simulink model "SF049A_LoaMgr"  (R2013b)
settings: Solver=FixedStepDiscrete  SolverMode=SingleTasking  StartTime=0.0  StopTime=1  FixedStep=0.002  RelTol=1e-3
values from neighbouring files (symbols this model uses):
  CURRMEASLOAMTGTNMASK_CNT_U08 = DataDict.Constant    [SF049A_LoaMgr_DataDict.m]
  IVTRLOAMTGTNMASK_CNT_U08 = DataDict.Constant    [SF049A_LoaMgr_DataDict.m]
  LOAMAXSLEW_ULSPERSEC_F32 = DataDict.Constant    [SF049A_LoaMgr_DataDict.m]
  LoaMgrCurrIvtrMtgtnRate = DataDict.Calibration    [SF049A_LoaMgr_DataDict.m]
  LoaMgrCurrIvtrMtgtnSca = DataDict.Calibration    [SF049A_LoaMgr_DataDict.m]
  LoaMgrCurrIvtrMtgtnScaZeroEna = DataDict.Calibration    [SF049A_LoaMgr_DataDict.m]
  LoaMgrCurrMeasIdptSig0Resp = DataDict.Calibration    [SF049A_LoaMgr_DataDict.m]
  LoaMgrCurrMeasIdptSig1Resp = DataDict.Calibration    [SF049A_LoaMgr_DataDict.m]
  LoaMgrCurrMeasIdptSig2Resp = DataDict.Calibration    [SF049A_LoaMgr_DataDict.m]
  LoaMgrCurrMeasIdptSigFltThd = DataDict.Calibration    [SF049A_LoaMgr_DataDict.m]
  LoaMgrCurrMeasMtgtnRate = DataDict.Calibration    [SF049A_LoaMgr_DataDict.m]
  LoaMgrCurrMeasMtgtnSca = DataDict.Calibration    [SF049A_LoaMgr_DataDict.m]
  LoaMgrCurrMeasMtgtnScaZeroEna = DataDict.Calibration    [SF049A_LoaMgr_DataDict.m]
  LoaMgrFadeOutStRate = DataDict.Calibration    [SF049A_LoaMgr_DataDict.m]
  LoaMgrHwTqIdptSig0NoTqLoaResp = DataDict.Calibration    [SF049A_LoaMgr_DataDict.m]
  LoaMgrHwTqIdptSig1NoTqLoaResp = DataDict.Calibration    [SF049A_LoaMgr_DataDict.m]
  LoaMgrHwTqIdptSig2Resp = DataDict.Calibration    [SF049A_LoaMgr_DataDict.m]
  LoaMgrHwTqIdptSig4Resp = DataDict.Calibration    [SF049A_LoaMgr_DataDict.m]
  LoaMgrHwTqIdptSigFltThd = DataDict.Calibration    [SF049A_LoaMgr_DataDict.m]
  LoaMgrHwTqLoaAvlResp = DataDict.Calibration    [SF049A_LoaMgr_DataDict.m]
  LoaMgrIvtrIdptSig0Resp = DataDict.Calibration    [SF049A_LoaMgr_DataDict.m]
  LoaMgrIvtrIdptSig1Resp = DataDict.Calibration    [SF049A_LoaMgr_DataDict.m]
  LoaMgrIvtrIdptSig2Resp = DataDict.Calibration    [SF049A_LoaMgr_DataDict.m]
  LoaMgrIvtrIdptSigFltThd = DataDict.Calibration    [SF049A_LoaMgr_DataDict.m]
  LoaMgrIvtrMtgtnRate = DataDict.Calibration    [SF049A_LoaMgr_DataDict.m]
  LoaMgrIvtrMtgtnSca = DataDict.Calibration    [SF049A_LoaMgr_DataDict.m]
  LoaMgrIvtrMtgtnScaZeroEna = DataDict.Calibration    [SF049A_LoaMgr_DataDict.m]
  LoaMgrLimdStRate = DataDict.Calibration    [SF049A_LoaMgr_DataDict.m]
  LoaMgrLimdStSca = DataDict.Calibration    [SF049A_LoaMgr_DataDict.m]
  LoaMgrMotAgAvlSnsrlsResp = DataDict.Calibration    [SF049A_LoaMgr_DataDict.m]
  LoaMgrMotAgIdptSig0NoSnsrlsResp = DataDict.Calibration    [SF049A_LoaMgr_DataDict.m]
  LoaMgrMotAgIdptSig1NoSnsrlsResp = DataDict.Calibration    [SF049A_LoaMgr_DataDict.m]
  LoaMgrMotAgIdptSig2Resp = DataDict.Calibration    [SF049A_LoaMgr_DataDict.m]
  LoaMgrMotAgIdptSig3Resp = DataDict.Calibration    [SF049A_LoaMgr_DataDict.m]
  LoaMgrMotAgIdptSigFltThd = DataDict.Calibration    [SF049A_LoaMgr_DataDict.m]
  LoaMgrMotAgMtgtnRate = DataDict.Calibration    [SF049A_LoaMgr_DataDict.m]
  LoaMgrMotAgMtgtnSca = DataDict.Calibration    [SF049A_LoaMgr_DataDict.m]
  LoaMgrMotAgMtgtnScaZeroEna = DataDict.Calibration    [SF049A_LoaMgr_DataDict.m]
  LOASCAONE_ULS_F32 = DataDict.Constant    [SF049A_LoaMgr_DataDict.m]
  LOASCAZERO_ULS_F32 = DataDict.Constant    [SF049A_LoaMgr_DataDict.m]
  LOASTIMDTSHTDWN_CNT_U08 = DataDict.Constant    [SF049A_LoaMgr_DataDict.m]
  LOASTNORM_CNT_U08 = DataDict.Constant    [SF049A_LoaMgr_DataDict.m]
  LOASTSWMTGTN_CNT_U08 = DataDict.Constant    [SF049A_LoaMgr_DataDict.m]
  MAXCURRMEASIDPTSIGALLWD_CNT_U08 = DataDict.Constant    [SF049A_LoaMgr_DataDict.m]
  MAXHWTQIDPTSIGALLWD_CNT_U08 = DataDict.Constant    [SF049A_LoaMgr_DataDict.m]
  MAXIVTRIDPTSIGALLWD_CNT_U08 = DataDict.Constant    [SF049A_LoaMgr_DataDict.m]
  MAXMOTAGMECLIDPTSIGALLWD_CNT_U08 = DataDict.Constant    [SF049A_LoaMgr_DataDict.m]
  NODEBSTEP_CNT_U16 = DataDict.Constant    [SF049A_LoaMgr_DataDict.m]
undefined symbols (not defined in the file or in its folder): LoaSt1, NtcNr1, NtcSts1, SigQlfr1
libraries: simulink x43, NxtrMin x4, NxtrMax x4, NxtrLim x2
(part 5 of 8)

== system SF049A_LoaMgr/LoaMgr/LoaMgrPer1/Request_Responses/InvtrResp ==
  note: SWITCH IvtrIdptMin
      |     CASE 2
      |         CurrMeasResp = LoaMgrIvtrIdptSig2Resp
      |     CASE 1
      |          CurrMeasResp = LoaMgrIvtrIdptSig1Resp
      |     CASE ELSE
      |          CurrMeasResp = LoaMgrIvtrIdptSig0Resp
      | ENDSWITCH
  IvtrIdptMin : Inport  RequirementInfo="{'linktype_rmi_doors' '0000bab3 (/E-STEER Core/SubSystem Specifications/Application Functions/SF049A Loss of Assist Manager)' '#SF049A_65' 'true' 'REQ:  SF049A_65' '' } %GIDa_1b89cce5_9f06_4c0e_ba65_24a38e656f3b"
  Constant : Constant  RequirementInfo="{'linktype_rmi_doors' '0000bab3 (/E-STEER Core/SubSystem Specifications/Application Functions/SF049A Loss of Assist Manager)' '#SF049A_65' 'true' 'REQ:  SF049A_65' '' } %GIDa_4fe7916c_bbcd_4978_b0d8_6de832c7292f"  Value=LoaMgrIvtrIdptSig2Resp
  Constant1 : Constant  RequirementInfo="{'linktype_rmi_doors' '0000bab3 (/E-STEER Core/SubSystem Specifications/Application Functions/SF049A Loss of Assist Manager)' '#SF049A_65' 'true' 'REQ:  SF049A_65' '' } %GIDa_0bdb73f6_8162_4fab_b11a_dceccb5a49a9"  Value=LoaMgrIvtrIdptSig1Resp
  Constant2 : Constant  RequirementInfo="{'linktype_rmi_doors' '0000bab3 (/E-STEER Core/SubSystem Specifications/Application Functions/SF049A Loss of Assist Manager)' '#SF049A_65' 'true' 'REQ:  SF049A_65' '' } %GIDa_9cb0bfe4_9355_407e_8f9d_9d090e8a3b93"  Value=LoaMgrIvtrIdptSig0Resp
  CopyRight2 : Subsystem  Description=|  mask(Copyright Information){none=on}
      | Copyright info block.                                               
      |                                                                     
      | Place copyright information at the top of every subsystem in design.
      mask prompts: none "No parameters"
      mask help: Place copyright information at the top of every subsystem in design.
      mask Display:
      | NxtrConf = 'Nexteer Confidential';
      | 
      | sys = bdroot; %handle for the current model ("system")
      | first = get_param(sys,'Created');
      | first = first(end-3:end);  %year is last four digits
      | 
      | last = get_param(sys,'LastModifiedDate');
      | if isempty(last)
      |     last = datestr(now,'yyyy');
      | else
      |     last = last(end-3:end);
      | end
      | 
      | if strcmp(first,last)
      |     fprintf('%s -- Copyright %s Nexteer',NxtrConf,first)
      | else
      |     fprintf('%s -- %s%s- %s Nexteer',NxtrConf,char(169),first,last)
      | end
  Merge1 : Merge  RequirementInfo="{'linktype_rmi_doors' '0000bab3 (/E-STEER Core/SubSystem Specifications/Application Functions/SF049A Loss of Assist Manager)' '#SF049A_65' 'true' 'REQ:  SF049A_65' '' } %GIDa_53806811_0184_454b_a74e_b9ca97a7c082"  Inputs=3
  Switch Case : SwitchCase  RequirementInfo="{'linktype_rmi_doors' '0000bab3 (/E-STEER Core/SubSystem Specifications/Application Functions/SF049A Loss of Assist Manager)' '#SF049A_65' 'true' 'REQ:  SF049A_65' '' } %GIDa_b306f5cf_a607_4f83_8634_b627f8551966"  CaseConditions={2,1}
  Two : Subsystem  RequirementInfo="{'linktype_rmi_doors' '0000bab3 (/E-STEER Core/SubSystem Specifications/Application Functions/SF049A Loss of Assist Manager)' '#SF049A_65' 'true' 'REQ:  SF049A_65' '' } %GIDa_33864284_e6bd_4345_a4a1_34ef31650c1d"  TreatAsAtomicUnit=on
      settings: RTWSystemCode=Inline
  Zero_or_Invalid : Subsystem  RequirementInfo="{'linktype_rmi_doors' '0000bab3 (/E-STEER Core/SubSystem Specifications/Application Functions/SF049A Loss of Assist Manager)' '#SF049A_65' 'true' 'REQ:  SF049A_65' '' } %GIDa_401ac225_c869_4784_ab56_815fb2158ee0"  TreatAsAtomicUnit=on
      settings: RTWSystemCode=Inline
  one : Subsystem  RequirementInfo="{'linktype_rmi_doors' '0000bab3 (/E-STEER Core/SubSystem Specifications/Application Functions/SF049A Loss of Assist Manager)' '#SF049A_65' 'true' 'REQ:  SF049A_65' '' } %GIDa_12453c58_6b24_4675_9de5_6df473c66688"  TreatAsAtomicUnit=on
      settings: RTWSystemCode=Inline
  IvtrResp : Outport  RequirementInfo="{'linktype_rmi_doors' '0000bab3 (/E-STEER Core/SubSystem Specifications/Application Functions/SF049A Loss of Assist Manager)' '#SF049A_65' 'true' 'REQ:  SF049A_65' '' } %GIDa_419d50e3_e95b_423c_91ee_694b6f829bad"
  wires:
  Constant2/1 -> Zero_or_Invalid/1(Sig0Resp)
  Zero_or_Invalid/1(IvtrResp) -> Merge1/3
  Merge1/1 -> IvtrResp/1
  one/1(IvtrResp) -> Merge1/2
  Two/1(IvtrResp) -> Merge1/1
  Constant1/1 -> one/1(Sig1Resp)
  Switch Case/2 -> one/Action
  Constant/1 -> Two/1(Sig2Resp)
  Switch Case/1 -> Two/Action
  Switch Case/3 -> Zero_or_Invalid/Action
  IvtrIdptMin/1 -> Switch Case/1

== system SF049A_LoaMgr/LoaMgr/LoaMgrPer1/Request_Responses/MotAgResp ==
  note: SWITCH MotPosnActvMin
      |     CASE 3
      |         MotAgResp = LoaMgrMotAgIdptSig3Resp
      |     CASE 2
      |         MotAgResp = LoaMgrMotAgIdptSig2Resp
      |     CASE 1
      |         IF SnsrlsMotAgAvl == true
      |             MotAgResp = LoaMgrMotAgAvlSnsrlsResp
      |         ELSE
      |             MotAgResp = LoaMgrMotAgIdptSig1NoSnsrlsResp
      |         ENDIF
      |     CASE ELSE
      |         IF SnsrlsMotAgAvl == true
      |             MotAgResp = LoaMgrMotAgAvlSnsrlsResp
      |         ELSE
      |             MotAgResp = LoaMgrMotAgIdptSig0NoSnsrlsResp
      |         ENDIF
      | ENDSWITCH
  MotAgIdptMin : Inport
  MotAgAvlSnsrls : Inport  Port=2
  Constant : Constant  RequirementInfo="{'linktype_rmi_doors' '0000bab3 (/E-STEER Core/SubSystem Specifications/Application Functions/SF049A Loss of Assist Manager)' '#SF049A_62' 'true' 'REQ:  SF049A_62' '' } %GIDa_fe7df534_0d0e_4361_a7d1_8d990e9503fd"  Value=LoaMgrMotAgIdptSig3Resp
  Constant1 : Constant  RequirementInfo="{'linktype_rmi_doors' '0000bab3 (/E-STEER Core/SubSystem Specifications/Application Functions/SF049A Loss of Assist Manager)' '#SF049A_62' 'true' 'REQ:  SF049A_62' '' } %GIDa_3d9c6392_b13d_4a1b_b0fc_24f927be1f2e"  Value=LoaMgrMotAgIdptSig2Resp
  Constant2 : Constant  RequirementInfo="{'linktype_rmi_doors' '0000bab3 (/E-STEER Core/SubSystem Specifications/Application Functions/SF049A Loss of Assist Manager)' '#SF049A_62' 'true' 'REQ:  SF049A_62' '' } %GIDa_0f6f8213_e738_43db_a6c9_e00157f70c62"  Value=LoaMgrMotAgAvlSnsrlsResp
  Constant3 : Constant  RequirementInfo="{'linktype_rmi_doors' '0000bab3 (/E-STEER Core/SubSystem Specifications/Application Functions/SF049A Loss of Assist Manager)' '#SF049A_62' 'true' 'REQ:  SF049A_62' '' } %GIDa_41dc0631_0cc8_4d4c_af56_d92212e830e8"  Value=LoaMgrMotAgIdptSig1NoSnsrlsResp
  Constant4 : Constant  RequirementInfo="{'linktype_rmi_doors' '0000bab3 (/E-STEER Core/SubSystem Specifications/Application Functions/SF049A Loss of Assist Manager)' '#SF049A_62' 'true' 'REQ:  SF049A_62' '' } %GIDa_a9758e5d_db59_4e76_b72d_8b72399f1ee9"  Value=LoaMgrMotAgAvlSnsrlsResp
  Constant5 : Constant  RequirementInfo="{'linktype_rmi_doors' '0000bab3 (/E-STEER Core/SubSystem Specifications/Application Functions/SF049A Loss of Assist Manager)' '#SF049A_62' 'true' 'REQ:  SF049A_62' '' } %GIDa_35d7b4b3_9a97_4d0f_8c9e_f031fc83a105"  Value=LoaMgrMotAgIdptSig0NoSnsrlsResp
  CopyRight2 : Subsystem  Description=|  mask(Copyright Information){none=on}
      | Copyright info block.                                               
      |                                                                     
      | Place copyright information at the top of every subsystem in design.
      mask prompts: none "No parameters"
      mask help: Place copyright information at the top of every subsystem in design.
      mask Display:
      | NxtrConf = 'Nexteer Confidential';
      | 
      | sys = bdroot; %handle for the current model ("system")
      | first = get_param(sys,'Created');
      | first = first(end-3:end);  %year is last four digits
      | 
      | last = get_param(sys,'LastModifiedDate');
      | if isempty(last)
      |     last = datestr(now,'yyyy');
      | else
      |     last = last(end-3:end);
      | end
      | 
      | if strcmp(first,last)
      |     fprintf('%s -- Copyright %s Nexteer',NxtrConf,first)
      | else
      |     fprintf('%s -- %s%s- %s Nexteer',NxtrConf,char(169),first,last)
      | end
  Merge1 : Merge  RequirementInfo="{'linktype_rmi_doors' '0000bab3 (/E-STEER Core/SubSystem Specifications/Application Functions/SF049A Loss of Assist Manager)' '#SF049A_62' 'true' 'REQ:  SF049A_62' '' } %GIDa_f74c0f8f_6199_42c9_a9b4_9fe75ac279f8"  Inputs=4
  Switch Case : SwitchCase  RequirementInfo="{'linktype_rmi_doors' '0000bab3 (/E-STEER Core/SubSystem Specifications/Application Functions/SF049A Loss of Assist Manager)' '#SF049A_62' 'true' 'REQ:  SF049A_62' '' } %GIDa_a503ffae_3f7c_4ab2_ac8d_b3698489ab48"  CaseConditions={3,2,1}
  Three : Subsystem  RequirementInfo="{'linktype_rmi_doors' '0000bab3 (/E-STEER Core/SubSystem Specifications/Application Functions/SF049A Loss of Assist Manager)' '#SF049A_62' 'true' 'REQ:  SF049A_62' '' } %GIDa_4f2af8ad_7a80_4958_bbd0_800287e60209"  TreatAsAtomicUnit=on
      settings: RTWSystemCode=Inline
  Two : Subsystem  RequirementInfo="{'linktype_rmi_doors' '0000bab3 (/E-STEER Core/SubSystem Specifications/Application Functions/SF049A Loss of Assist Manager)' '#SF049A_62' 'true' 'REQ:  SF049A_62' '' } %GIDa_1d288f99_f817_4baa_9517_46b598207607"  TreatAsAtomicUnit=on
      settings: RTWSystemCode=Inline
  Zero_or_Invalid : Subsystem  RequirementInfo="{'linktype_rmi_doors' '0000bab3 (/E-STEER Core/SubSystem Specifications/Application Functions/SF049A Loss of Assist Manager)' '#SF049A_62' 'true' 'REQ:  SF049A_62' '' } %GIDa_acdb447e_c366_4a14_b525_2a008c13cd34"  TreatAsAtomicUnit=on
      settings: RTWSystemCode=Inline
  one : Subsystem  RequirementInfo="{'linktype_rmi_doors' '0000bab3 (/E-STEER Core/SubSystem Specifications/Application Functions/SF049A Loss of Assist Manager)' '#SF049A_62' 'true' 'REQ:  SF049A_62' '' } %GIDa_0c344591_bf08_46ad_8169_64860ee94572"  TreatAsAtomicUnit=on
      settings: RTWSystemCode=Inline
  MotAgResp : Outport  RequirementInfo={} %GIDa_7b82afc9_717d_4b23_8ce3_af9ce8de6a45
  wires:
  Merge1/1 -> MotAgResp/1
  Zero_or_Invalid/1(MotAgResp) -> Merge1/4
  one/1(MotAgResp) -> Merge1/3
  Two/1(MotAgResp) -> Merge1/2
  Three/1(MotAgResp) -> Merge1/1
  [MotAgAvlSnsrls] -> Zero_or_Invalid/3(MotAgAvlSnsrls)
  Constant5/1 -> Zero_or_Invalid/2(MotAgIdptSig0NoResp)
  Constant4/1 -> Zero_or_Invalid/1(MotAgAvlSnsrlsResp)
  [MotAgAvlSnsrls] -> one/3(MotAgAvlSnsrls)
  MotAgAvlSnsrls/1 -> [MotAgAvlSnsrls]
  Constant3/1 -> one/2(MotAgIdptSig1NoResp)
  Constant2/1 -> one/1(MotAgAvlSnsrlsResp)
  Constant1/1 -> Two/1(cal)
  Switch Case/2 -> Two/Action
  Constant/1 -> Three/1(cal)
  Switch Case/1 -> Three/Action
  Switch Case/4 -> Zero_or_Invalid/Action
  MotAgIdptMin/1 -> Switch Case/1
  Switch Case/3 -> one/Action

== system SF049A_LoaMgr/LoaMgr/LoaMgrPer1/Set_Faults/CopyRight2 ==

== system SF049A_LoaMgr/LoaMgr/LoaMgrPer1/Set_Faults/NTC_Fault1 ==
  NtcNr : Inport
  NtcStInfo : Inport  Port=2
  NtcSts : Inport  Port=3
  DebStep : Inport  Port=4
  CallDiagMgr : ActionPort  ActionType=then
  SetNtcSts : Subsystem  RequirementInfo={} %GIDa_ec14747d_0fb9_427d_8c4c_05d0a3168c5b  TreatAsAtomicUnit=on
      settings: RTWSystemCode=Inline
  wires:
  NtcNr/1 -> SetNtcSts/1(NtcNr)  "NtcNr"
  NtcSts/1 -> SetNtcSts/3(NtcSts)
  DebStep/1 -> SetNtcSts/4(DebStep)
  NtcStInfo/1 -> SetNtcSts/2(NtcStInfo)

== system SF049A_LoaMgr/LoaMgr/LoaMgrPer1/Set_Faults/NTC_Fault2 ==
  NtcNr : Inport
  NtcStInfo : Inport  Port=2
  NtcSts : Inport  Port=3
  DebStep : Inport  Port=4
  CallDiagMgr : ActionPort  ActionType=elseif
  SetNtcSts : Subsystem  RequirementInfo={} %GIDa_0314a1a3_06fe_40a3_8d28_9216caabfc6d  TreatAsAtomicUnit=on
      settings: RTWSystemCode=Inline
  wires:
  NtcStInfo/1 -> SetNtcSts/2(NtcStInfo)
  DebStep/1 -> SetNtcSts/4(DebStep)
  NtcSts/1 -> SetNtcSts/3(NtcSts)
  NtcNr/1 -> SetNtcSts/1(NtcNr)  "NtcNr"

== system SF049A_LoaMgr/LoaMgr/LoaMgrPer1/Set_Faults/NTC_Fault3 ==
  NtcNr : Inport
  NtcStInfo : Inport  Port=2
  NtcSts : Inport  Port=3
  DebStep : Inport  Port=4
  CallDiagMgr : ActionPort  ActionType=then
  SetNtcSts : Subsystem  RequirementInfo={} %GIDa_0554f703_9e04_463e_b1df_1878644cbe3a  TreatAsAtomicUnit=on
      settings: RTWSystemCode=Inline
  wires:
  NtcStInfo/1 -> SetNtcSts/2(NtcStInfo)
  DebStep/1 -> SetNtcSts/4(DebStep)
  NtcSts/1 -> SetNtcSts/3(NtcSts)
  NtcNr/1 -> SetNtcSts/1(NtcNr)  "NtcNr"

== system SF049A_LoaMgr/LoaMgr/LoaMgrPer1/Set_Faults/NTC_Fault4 ==
  NtcNr : Inport
  NtcStInfo : Inport  Port=2
  NtcSts : Inport  Port=3
  DebStep : Inport  Port=4
  CallDiagMgr : ActionPort  ActionType=then
  SetNtcSts : Subsystem  RequirementInfo={} %GIDa_e6206b51_9847_4131_8871_117a3d33ca7a  TreatAsAtomicUnit=on
      settings: RTWSystemCode=Inline
  wires:
  NtcNr/1 -> SetNtcSts/1(NtcNr)  "NtcNr"
  NtcSts/1 -> SetNtcSts/3(NtcSts)
  DebStep/1 -> SetNtcSts/4(DebStep)
  NtcStInfo/1 -> SetNtcSts/2(NtcStInfo)

== system SF049A_LoaMgr/LoaMgr/LoaMgrPer1/Set_Faults/NTC_Fault5 ==
  NtcNr : Inport
  NtcStInfo : Inport  Port=2
  NtcSts : Inport  Port=3
  DebStep : Inport  Port=4
  CallDiagMgr : ActionPort  ActionType=then
  CopyRight2 : Subsystem  Description=|  mask(Copyright Information){none=on}
      | Copyright info block.                                               
      |                                                                     
      | Place copyright information at the top of every subsystem in design.
      mask prompts: none "No parameters"
      mask help: Place copyright information at the top of every subsystem in design.
      mask Display:
      | NxtrConf = 'Nexteer Confidential';
      | 
      | sys = bdroot; %handle for the current model ("system")
      | first = get_param(sys,'Created');
      | first = first(end-3:end);  %year is last four digits
      | 
      | last = get_param(sys,'LastModifiedDate');
      | if isempty(last)
      |     last = datestr(now,'yyyy');
      | else
      |     last = last(end-3:end);
      | end
      | 
      | if strcmp(first,last)
      |     fprintf('%s -- Copyright %s Nexteer',NxtrConf,first)
      | else
      |     fprintf('%s -- %s%s- %s Nexteer',NxtrConf,char(169),first,last)
      | end
  Data Store Write1 : DataStoreWrite  DataStoreName=DebStep
  Data Store Write3 : DataStoreWrite  DataStoreName=Fault5_Status
  Terminator : Terminator
  Terminator1 : Terminator
  wires:
  NtcStInfo/1 -> Terminator1/1
  DebStep/1 -> Data Store Write1/1
  NtcSts/1 -> Data Store Write3/1
  NtcNr/1 -> Terminator/1

== system SF049A_LoaMgr/LoaMgr/LoaMgrPer1/Set_Faults/NTC_Fault6 ==
  NtcNr : Inport
  NtcStInfo : Inport  Port=2
  NtcSts : Inport  Port=3
  DebStep : Inport  Port=4
  CallDiagMgr : ActionPort  ActionType=then
  CopyRight2 : Subsystem  Description=|  mask(Copyright Information){none=on}
      | Copyright info block.                                               
      |                                                                     
      | Place copyright information at the top of every subsystem in design.
      mask prompts: none "No parameters"
      mask help: Place copyright information at the top of every subsystem in design.
      mask Display:
      | NxtrConf = 'Nexteer Confidential';
      | 
      | sys = bdroot; %handle for the current model ("system")
      | first = get_param(sys,'Created');
      | first = first(end-3:end);  %year is last four digits
      | 
      | last = get_param(sys,'LastModifiedDate');
      | if isempty(last)
      |     last = datestr(now,'yyyy');
      | else
      |     last = last(end-3:end);
      | end
      | 
      | if strcmp(first,last)
      |     fprintf('%s -- Copyright %s Nexteer',NxtrConf,first)
      | else
      |     fprintf('%s -- %s%s- %s Nexteer',NxtrConf,char(169),first,last)
      | end
  Data Store Write1 : DataStoreWrite  DataStoreName=DebStep
  Data Store Write3 : DataStoreWrite  DataStoreName=Fault6_Status
  Terminator : Terminator
  Terminator1 : Terminator
  wires:
  NtcNr/1 -> Terminator/1
  NtcSts/1 -> Data Store Write3/1
  DebStep/1 -> Data Store Write1/1
  NtcStInfo/1 -> Terminator1/1

== system SF049A_LoaMgr/ISO Fault Debounce/DiagMgr/NTCSTS_PREFAILD/If Action Subsystem1/CopyRight2 ==

== system SF049A_LoaMgr/ISO Fault Debounce/DiagMgr/NTCSTS_PREFAILD/If Action Subsystem1/If Action Subsystem ==
  EA : Inport
  Qlf : Inport  Port=2
  Action Port : ActionPort  ActionType=then
  EAo : Outport
  Qlfo : Outport  Port=2
  wires:
  EA/1 -> EAo/1
  Qlf/1 -> Qlfo/1

== system SF049A_LoaMgr/ISO Fault Debounce/DiagMgr/NTCSTS_PREFAILD/If Action Subsystem1/If Action Subsystem1 ==
  EA : Inport
  Qlf : Inport  Port=2
  Action Port : ActionPort  ActionType=else
  EAo : Outport
  Qlfo : Outport  Port=2
  wires:
  EA/1 -> EAo/1
  Qlf/1 -> Qlfo/1

== system SF049A_LoaMgr/LoaMgr/LoaMgrInit1/NTC_Fault1/SetNtcSts/CopyRight2 ==

== system SF049A_LoaMgr/LoaMgr/LoaMgrInit1/NTC_Fault2/SetNtcSts/CopyRight2 ==

== system SF049A_LoaMgr/LoaMgr/LoaMgrInit1/NTC_Fault3/SetNtcSts/CopyRight2 ==

== system SF049A_LoaMgr/LoaMgr/LoaMgrInit1/NTC_Fault4/SetNtcSts/CopyRight2 ==

== system SF049A_LoaMgr/LoaMgr/LoaMgrInit1/NTC_Fault5/SetNtcSts/CopyRight2 ==

== system SF049A_LoaMgr/LoaMgr/LoaMgrInit1/NTC_Fault6/SetNtcSts/CopyRight2 ==

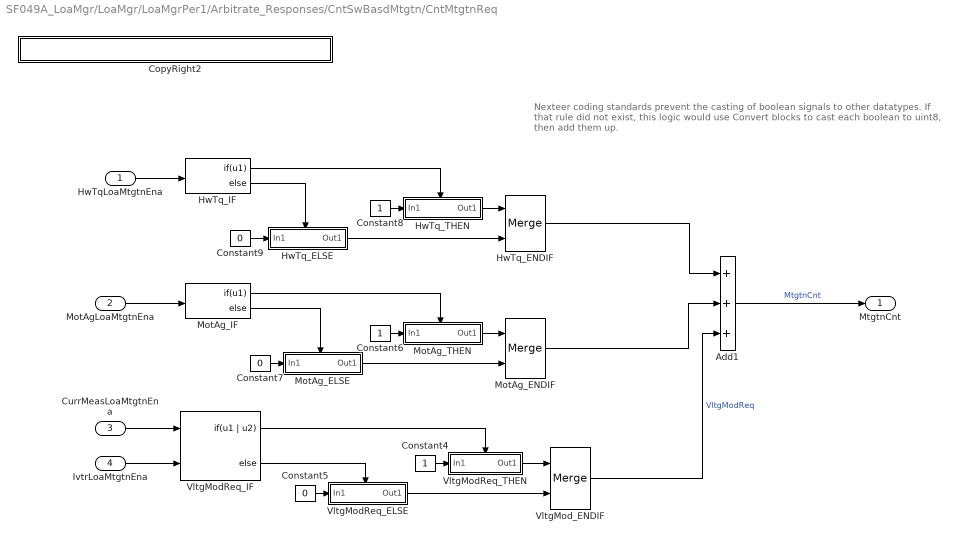
== system SF049A_LoaMgr/LoaMgr/LoaMgrPer1/Arbitrate_Responses/CntSwBasdMtgtn/CntMtgtnReq ==
  note: Nexteer coding standards prevent the casting of boolean signals to other datatypes.
      | If that rule did not exist, this logic would use Convert blocks to cast each boolean
      | to uint8, then add them up.
  HwTqLoaMtgtnEna : Inport  RequirementInfo="{'linktype_rmi_doors' '0000bab3 (/E-STEER Core/SubSystem Specifications/Application Functions/SF049A Loss of Assist Manager)' '#SF049A_79' 'true' 'REQ:  SF049A_79' '' } %GIDa_daf9ec58_ac26_46ac_a144_d220a5a763f7"
  MotAgLoaMtgtnEna : Inport  RequirementInfo="{'linktype_rmi_doors' '0000bab3 (/E-STEER Core/SubSystem Specifications/Application Functions/SF049A Loss of Assist Manager)' '#SF049A_79' 'true' 'REQ:  SF049A_79' '' } %GIDa_297248ed_ee1c_47d4_ae0d_18f5b1e6cdaf"  Port=2
  CurrMeasLoaMtgtnEna : Inport  RequirementInfo="{'linktype_rmi_doors' '0000bab3 (/E-STEER Core/SubSystem Specifications/Application Functions/SF049A Loss of Assist Manager)' '#SF049A_78' 'true' 'REQ:  SF049A_78' '' } %GIDa_c4583923_c377_45c9_a212_6d953514ef30"  Port=3
  IvtrLoaMtgtnEna : Inport  RequirementInfo="{'linktype_rmi_doors' '0000bab3 (/E-STEER Core/SubSystem Specifications/Application Functions/SF049A Loss of Assist Manager)' '#SF049A_78' 'true' 'REQ:  SF049A_78' '' } %GIDa_26d1a7f8_3650_4109_85b3_a63a6fdfbb70"  Port=4
  Add1 : Sum  RequirementInfo="{'linktype_rmi_doors' '0000bab3 (/E-STEER Core/SubSystem Specifications/Application Functions/SF049A Loss of Assist Manager)' '#SF049A_79' 'true' 'REQ:  SF049A_79' '' } %GIDa_e056b890_f6f5_421f_8c34_7cd2f00d2b44"  Inputs=+++
  Constant4 : Constant  RequirementInfo="{'linktype_rmi_doors' '0000bab3 (/E-STEER Core/SubSystem Specifications/Application Functions/SF049A Loss of Assist Manager)' '#SF049A_78' 'true' 'REQ:  SF049A_78' '' } %GIDa_653efff9_ef9c_4773_9856_96f77ea5374d"  OutDataTypeStr=uint8
      settings: AttributesFormatString=%<OutDataTypeStr>
  Constant5 : Constant  RequirementInfo="{'linktype_rmi_doors' '0000bab3 (/E-STEER Core/SubSystem Specifications/Application Functions/SF049A Loss of Assist Manager)' '#SF049A_78' 'true' 'REQ:  SF049A_78' '' } %GIDa_9496bbb8_1dbd_4b40_a324_67c0f76ade5d"  Value=0  OutDataTypeStr=uint8
      settings: AttributesFormatString=%<OutDataTypeStr>
  Constant6 : Constant  RequirementInfo="{'linktype_rmi_doors' '0000bab3 (/E-STEER Core/SubSystem Specifications/Application Functions/SF049A Loss of Assist Manager)' '#SF049A_79' 'true' 'REQ:  SF049A_79' '' } %GIDa_b2ad5597_a9fa_4d2b_9588_92e994b86849"  OutDataTypeStr=uint8
      settings: AttributesFormatString=%<OutDataTypeStr>
  Constant7 : Constant  RequirementInfo="{'linktype_rmi_doors' '0000bab3 (/E-STEER Core/SubSystem Specifications/Application Functions/SF049A Loss of Assist Manager)' '#SF049A_79' 'true' 'REQ:  SF049A_79' '' } %GIDa_a1a1dc4e_b570_402e_9cbb_69849cd808ae"  Value=0  OutDataTypeStr=uint8
      settings: AttributesFormatString=%<OutDataTypeStr>
  Constant8 : Constant  RequirementInfo="{'linktype_rmi_doors' '0000bab3 (/E-STEER Core/SubSystem Specifications/Application Functions/SF049A Loss of Assist Manager)' '#SF049A_79' 'true' 'REQ:  SF049A_79' '' } %GIDa_f6dd6a9d_9ad6_478f_8362_ca4fc6facd58"  OutDataTypeStr=uint8
      settings: AttributesFormatString=%<OutDataTypeStr>
  Constant9 : Constant  RequirementInfo="{'linktype_rmi_doors' '0000bab3 (/E-STEER Core/SubSystem Specifications/Application Functions/SF049A Loss of Assist Manager)' '#SF049A_79' 'true' 'REQ:  SF049A_79' '' } %GIDa_e60b9b0f_1ab3_4bd3_935a_37e1dfb4b77e"  Value=0  OutDataTypeStr=uint8
      settings: AttributesFormatString=%<OutDataTypeStr>
  CopyRight2 : Subsystem  Description=|  mask(Copyright Information){none=on}
      | Copyright info block.                                               
      |                                                                     
      | Place copyright information at the top of every subsystem in design.
      mask prompts: none "No parameters"
      mask help: Place copyright information at the top of every subsystem in design.
      mask Display:
      | NxtrConf = 'Nexteer Confidential';
      | 
      | sys = bdroot; %handle for the current model ("system")
      | first = get_param(sys,'Created');
      | first = first(end-3:end);  %year is last four digits
      | 
      | last = get_param(sys,'LastModifiedDate');
      | if isempty(last)
      |     last = datestr(now,'yyyy');
      | else
      |     last = last(end-3:end);
      | end
      | 
      | if strcmp(first,last)
      |     fprintf('%s -- Copyright %s Nexteer',NxtrConf,first)
      | else
      |     fprintf('%s -- %s%s- %s Nexteer',NxtrConf,char(169),first,last)
      | end
  HwTq_ELSE : Subsystem  RequirementInfo="{'linktype_rmi_doors' '0000bab3 (/E-STEER Core/SubSystem Specifications/Application Functions/SF049A Loss of Assist Manager)' '#SF049A_79' 'true' 'REQ:  SF049A_79' '' } %GIDa_400e4d6a_ea92_4cca_ae02_575af306e939"  TreatAsAtomicUnit=on
      settings: RTWSystemCode=Inline
  HwTq_ENDIF : Merge  RequirementInfo="{'linktype_rmi_doors' '0000bab3 (/E-STEER Core/SubSystem Specifications/Application Functions/SF049A Loss of Assist Manager)' '#SF049A_79' 'true' 'REQ:  SF049A_79' '' } %GIDa_bb28ad8b_ef8c_48d5_bbbe_bc1fb55e1889"
  HwTq_IF : If  RequirementInfo="{'linktype_rmi_doors' '0000bab3 (/E-STEER Core/SubSystem Specifications/Application Functions/SF049A Loss of Assist Manager)' '#SF049A_79' 'true' 'REQ:  SF049A_79' '' } %GIDa_e0163281_2ded_47f9_b593_720f104bb3f3"  IfExpression=u1
  HwTq_THEN : Subsystem  RequirementInfo="{'linktype_rmi_doors' '0000bab3 (/E-STEER Core/SubSystem Specifications/Application Functions/SF049A Loss of Assist Manager)' '#SF049A_79' 'true' 'REQ:  SF049A_79' '' } %GIDa_2554efb7_f873_46e9_9a74_9f348ac7d7af"  TreatAsAtomicUnit=on
      settings: RTWSystemCode=Inline
  MotAg_ELSE : Subsystem  RequirementInfo="{'linktype_rmi_doors' '0000bab3 (/E-STEER Core/SubSystem Specifications/Application Functions/SF049A Loss of Assist Manager)' '#SF049A_79' 'true' 'REQ:  SF049A_79' '' } %GIDa_1ec685a6_c794_4bd9_a399_364b600a5a2d"  TreatAsAtomicUnit=on
      settings: RTWSystemCode=Inline
  MotAg_ENDIF : Merge  RequirementInfo="{'linktype_rmi_doors' '0000bab3 (/E-STEER Core/SubSystem Specifications/Application Functions/SF049A Loss of Assist Manager)' '#SF049A_79' 'true' 'REQ:  SF049A_79' '' } %GIDa_587bb4b2_1f9a_4db8_bdf8_6555dd9a50a7"
  MotAg_IF : If  RequirementInfo="{'linktype_rmi_doors' '0000bab3 (/E-STEER Core/SubSystem Specifications/Application Functions/SF049A Loss of Assist Manager)' '#SF049A_79' 'true' 'REQ:  SF049A_79' '' } %GIDa_630754a7_e444_4d93_ad54_324e3b07d7e8"  IfExpression=u1
  MotAg_THEN : Subsystem  RequirementInfo="{'linktype_rmi_doors' '0000bab3 (/E-STEER Core/SubSystem Specifications/Application Functions/SF049A Loss of Assist Manager)' '#SF049A_79' 'true' 'REQ:  SF049A_79' '' } %GIDa_89feefe6_ec0d_42d4_90dc_acc0ba3d6203"  TreatAsAtomicUnit=on
      settings: RTWSystemCode=Inline
  VltgModReq_ELSE : Subsystem  RequirementInfo="{'linktype_rmi_doors' '0000bab3 (/E-STEER Core/SubSystem Specifications/Application Functions/SF049A Loss of Assist Manager)' '#SF049A_78' 'true' 'REQ:  SF049A_78' '' } %GIDa_549f35d8_221d_4a1a_b106_ce719e3faf84"  TreatAsAtomicUnit=on
      settings: RTWSystemCode=Inline
  VltgModReq_IF : If  RequirementInfo="{'linktype_rmi_doors' '0000bab3 (/E-STEER Core/SubSystem Specifications/Application Functions/SF049A Loss of Assist Manager)' '#SF049A_78' 'true' 'REQ:  SF049A_78' '' } %GIDa_7c14cc30_e35c_41d0_9c65_a5bfd4288906"  NumInputs=2  IfExpression=u1 | u2
  VltgModReq_THEN : Subsystem  RequirementInfo="{'linktype_rmi_doors' '0000bab3 (/E-STEER Core/SubSystem Specifications/Application Functions/SF049A Loss of Assist Manager)' '#SF049A_78' 'true' 'REQ:  SF049A_78' '' } %GIDa_69e46b10_9737_4658_aa35_811bcd28dbe9"  TreatAsAtomicUnit=on
      settings: RTWSystemCode=Inline
  VltgMod_ENDIF : Merge  RequirementInfo="{'linktype_rmi_doors' '0000bab3 (/E-STEER Core/SubSystem Specifications/Application Functions/SF049A Loss of Assist Manager)' '#SF049A_78' 'true' 'REQ:  SF049A_78' '' ; 'linktype_rmi_doors' '0000bab3 (/E-STEER Core/SubSystem Specifications/Application Functions/SF049A Loss of Assist Manager)' '#SF049A_79' 'true' 'REQ:  SF049A_79' '' } %GIDa_716727ad_02a1_458f_be0d_953cf394e8e4"
  MtgtnCnt : Outport  RequirementInfo="{'linktype_rmi_doors' '0000bab3 (/E-STEER Core/SubSystem Specifications/Application Functions/SF049A Loss of Assist Manager)' '#SF049A_79' 'true' 'REQ:  SF049A_79' '' } %GIDa_52f63591_76c6_4960_af50_f09ccc098e28"
  wires:
  HwTqLoaMtgtnEna/1 -> HwTq_IF/1
  HwTq_ELSE/1(Out1) -> HwTq_ENDIF/2
  HwTq_THEN/1(Out1) -> HwTq_ENDIF/1
  Constant9/1 -> HwTq_ELSE/1(In1)
  Constant8/1 -> HwTq_THEN/1(In1)
  HwTq_IF/1 -> HwTq_THEN/Action
  HwTq_IF/2 -> HwTq_ELSE/Action
  MotAgLoaMtgtnEna/1 -> MotAg_IF/1
  MotAg_ELSE/1(Out1) -> MotAg_ENDIF/2
  MotAg_THEN/1(Out1) -> MotAg_ENDIF/1
  Constant7/1 -> MotAg_ELSE/1(In1)
  Constant6/1 -> MotAg_THEN/1(In1)
  MotAg_IF/1 -> MotAg_THEN/Action
  MotAg_IF/2 -> MotAg_ELSE/Action
  VltgModReq_ELSE/1(Out1) -> VltgMod_ENDIF/2
  VltgModReq_THEN/1(Out1) -> VltgMod_ENDIF/1
  Constant5/1 -> VltgModReq_ELSE/1(In1)
  Constant4/1 -> VltgModReq_THEN/1(In1)
  IvtrLoaMtgtnEna/1 -> VltgModReq_IF/2
  CurrMeasLoaMtgtnEna/1 -> VltgModReq_IF/1
  MotAg_ENDIF/1 -> Add1/2
  HwTq_ENDIF/1 -> Add1/1
  Add1/1 -> MtgtnCnt/1  "MtgtnCnt"
  VltgMod_ENDIF/1 -> Add1/3  "VltgModReq"
  VltgModReq_IF/1 -> VltgModReq_THEN/Action
  VltgModReq_IF/2 -> VltgModReq_ELSE/Action

== system SF049A_LoaMgr/LoaMgr/LoaMgrPer1/Arbitrate_Responses/CntSwBasdMtgtn/CopyRight2 ==

== system SF049A_LoaMgr/LoaMgr/LoaMgrPer1/Arbitrate_Responses/CntSwBasdMtgtn/IllegalCombination ==
  note: Early drafts of this design used a calibration here.  Peer review team
      | preferred to hardcode an Immediate Shutdown until customer requirements
      | become more clear.
  Action Port : ActionPort  ActionType=else
  Constant2 : Constant  RequirementInfo="{'linktype_rmi_doors' '0000bab3 (/E-STEER Core/SubSystem Specifications/Application Functions/SF049A Loss of Assist Manager)' '#SF049A_81' 'true' 'REQ:  SF049A_81' '' } %GIDa_d420531a_d9d3_465c_b19d_6885891660e6"  Value=LOASTIMDTSHTDWN_CNT_U08
  CopyRight2 : Subsystem  Description=|  mask(Copyright Information){none=on}
      | Copyright info block.                                               
      |                                                                     
      | Place copyright information at the top of every subsystem in design.
      mask prompts: none "No parameters"
      mask help: Place copyright information at the top of every subsystem in design.
      mask Display:
      | NxtrConf = 'Nexteer Confidential';
      | 
      | sys = bdroot; %handle for the current model ("system")
      | first = get_param(sys,'Created');
      | first = first(end-3:end);  %year is last four digits
      | 
      | last = get_param(sys,'LastModifiedDate');
      | if isempty(last)
      |     last = datestr(now,'yyyy');
      | else
      |     last = last(end-3:end);
      | end
      | 
      | if strcmp(first,last)
      |     fprintf('%s -- Copyright %s Nexteer',NxtrConf,first)
      | else
      |     fprintf('%s -- %s%s- %s Nexteer',NxtrConf,char(169),first,last)
      | end
  Out1 : Outport  RequirementInfo="{'linktype_rmi_doors' '0000bab3 (/E-STEER Core/SubSystem Specifications/Application Functions/SF049A Loss of Assist Manager)' '#SF049A_81' 'true' 'REQ:  SF049A_81' '' } %GIDa_97eec5b8_2ae8_4c62_b425_997f9fd78901"
  wires:
  Constant2/1 -> Out1/1

== system SF049A_LoaMgr/LoaMgr/LoaMgrPer1/Arbitrate_Responses/CntSwBasdMtgtn/OK_to_use ==
  Action Port : ActionPort  ActionType=then
  Constant : Constant  RequirementInfo="{'linktype_rmi_doors' '0000bab3 (/E-STEER Core/SubSystem Specifications/Application Functions/SF049A Loss of Assist Manager)' '#SF049A_81' 'true' 'REQ:  SF049A_81' '' } %GIDa_5a0dd816_c0c5_4127_811d_8acdf7880c3e"  Value=LOASTNORM_CNT_U08
  CopyRight2 : Subsystem  Description=|  mask(Copyright Information){none=on}
      | Copyright info block.                                               
      |                                                                     
      | Place copyright information at the top of every subsystem in design.
      mask prompts: none "No parameters"
      mask help: Place copyright information at the top of every subsystem in design.
      mask Display:
      | NxtrConf = 'Nexteer Confidential';
      | 
      | sys = bdroot; %handle for the current model ("system")
      | first = get_param(sys,'Created');
      | first = first(end-3:end);  %year is last four digits
      | 
      | last = get_param(sys,'LastModifiedDate');
      | if isempty(last)
      |     last = datestr(now,'yyyy');
      | else
      |     last = last(end-3:end);
      | end
      | 
      | if strcmp(first,last)
      |     fprintf('%s -- Copyright %s Nexteer',NxtrConf,first)
      | else
      |     fprintf('%s -- %s%s- %s Nexteer',NxtrConf,char(169),first,last)
      | end
  Out1 : Outport  RequirementInfo="{'linktype_rmi_doors' '0000bab3 (/E-STEER Core/SubSystem Specifications/Application Functions/SF049A Loss of Assist Manager)' '#SF049A_81' 'true' 'REQ:  SF049A_81' '' } %GIDa_b9a68fc4_e3e6_4297_85ab_3da976d4d777"
  wires:
  Constant/1 -> Out1/1

== system SF049A_LoaMgr/LoaMgr/LoaMgrPer1/Arbitrate_Responses/SelFinalResp/CopyRight2 ==

== system SF049A_LoaMgr/LoaMgr/LoaMgrPer1/Arbitrate_Responses/SelFinalResp/F1 ==
  F1 : ActionPort  ActionType=case
  CopyRight2 : Subsystem  Description=|  mask(Copyright Information){none=on}
      | Copyright info block.                                               
      |                                                                     
      | Place copyright information at the top of every subsystem in design.
      mask prompts: none "No parameters"
      mask help: Place copyright information at the top of every subsystem in design.
      mask Display:
      | NxtrConf = 'Nexteer Confidential';
      | 
      | sys = bdroot; %handle for the current model ("system")
      | first = get_param(sys,'Created');
      | first = first(end-3:end);  %year is last four digits
      | 
      | last = get_param(sys,'LastModifiedDate');
      | if isempty(last)
      |     last = datestr(now,'yyyy');
      | else
      |     last = last(end-3:end);
      | end
      | 
      | if strcmp(first,last)
      |     fprintf('%s -- Copyright %s Nexteer',NxtrConf,first)
      | else
      |     fprintf('%s -- %s%s- %s Nexteer',NxtrConf,char(169),first,last)
      | end
  Enumerated Constant : simulink/Sources/Enumerated Constant  OutDataTypeStr=Enum: LoaSt1  Value=LoaSt1.LOAST_IMDTSHTDWNREQD  SampleTime=inf
  LoaSt : Outport
  wires:
  Enumerated Constant/1 -> LoaSt/1

== system SF049A_LoaMgr/LoaMgr/LoaMgrPer1/Arbitrate_Responses/SelFinalResp/F2 ==
  F2 : ActionPort  ActionType=case
  CopyRight2 : Subsystem  Description=|  mask(Copyright Information){none=on}
      | Copyright info block.                                               
      |                                                                     
      | Place copyright information at the top of every subsystem in design.
      mask prompts: none "No parameters"
      mask help: Place copyright information at the top of every subsystem in design.
      mask Display:
      | NxtrConf = 'Nexteer Confidential';
      | 
      | sys = bdroot; %handle for the current model ("system")
      | first = get_param(sys,'Created');
      | first = first(end-3:end);  %year is last four digits
      | 
      | last = get_param(sys,'LastModifiedDate');
      | if isempty(last)
      |     last = datestr(now,'yyyy');
      | else
      |     last = last(end-3:end);
      | end
      | 
      | if strcmp(first,last)
      |     fprintf('%s -- Copyright %s Nexteer',NxtrConf,first)
      | else
      |     fprintf('%s -- %s%s- %s Nexteer',NxtrConf,char(169),first,last)
      | end
  Enumerated Constant : simulink/Sources/Enumerated Constant  OutDataTypeStr=Enum: LoaSt1  Value=LoaSt1.LOAST_CTRLDSHTDWNREQD  SampleTime=inf
  LoaSt : Outport
  wires:
  Enumerated Constant/1 -> LoaSt/1

== system SF049A_LoaMgr/LoaMgr/LoaMgrPer1/Arbitrate_Responses/SelFinalResp/Fade_Out ==
  F2 : ActionPort  ActionType=case
  CopyRight2 : Subsystem  Description=|  mask(Copyright Information){none=on}
      | Copyright info block.                                               
      |                                                                     
      | Place copyright information at the top of every subsystem in design.
      mask prompts: none "No parameters"
      mask help: Place copyright information at the top of every subsystem in design.
      mask Display:
      | NxtrConf = 'Nexteer Confidential';
      | 
      | sys = bdroot; %handle for the current model ("system")
      | first = get_param(sys,'Created');
      | first = first(end-3:end);  %year is last four digits
      | 
      | last = get_param(sys,'LastModifiedDate');
      | if isempty(last)
      |     last = datestr(now,'yyyy');
      | else
      |     last = last(end-3:end);
      | end
      | 
      | if strcmp(first,last)
      |     fprintf('%s -- Copyright %s Nexteer',NxtrConf,first)
      | else
      |     fprintf('%s -- %s%s- %s Nexteer',NxtrConf,char(169),first,last)
      | end
  Enumerated Constant : simulink/Sources/Enumerated Constant  OutDataTypeStr=Enum: LoaSt1  Value=LoaSt1.LOAST_FADEOUT  SampleTime=inf
  LoaSt : Outport
  wires:
  Enumerated Constant/1 -> LoaSt/1

== system SF049A_LoaMgr/LoaMgr/LoaMgrPer1/Arbitrate_Responses/SelFinalResp/Fade_Out1 ==
  F2 : ActionPort  ActionType=default
  CopyRight2 : Subsystem  Description=|  mask(Copyright Information){none=on}
      | Copyright info block.                                               
      |                                                                     
      | Place copyright information at the top of every subsystem in design.
      mask prompts: none "No parameters"
      mask help: Place copyright information at the top of every subsystem in design.
      mask Display:
      | NxtrConf = 'Nexteer Confidential';
      | 
      | sys = bdroot; %handle for the current model ("system")
      | first = get_param(sys,'Created');
      | first = first(end-3:end);  %year is last four digits
      | 
      | last = get_param(sys,'LastModifiedDate');
      | if isempty(last)
      |     last = datestr(now,'yyyy');
      | else
      |     last = last(end-3:end);
      | end
      | 
      | if strcmp(first,last)
      |     fprintf('%s -- Copyright %s Nexteer',NxtrConf,first)
      | else
      |     fprintf('%s -- %s%s- %s Nexteer',NxtrConf,char(169),first,last)
      | end
  Enumerated Constant : simulink/Sources/Enumerated Constant  OutDataTypeStr=Enum: LoaSt1  Value=LoaSt1.LOAST_FADEOUT  SampleTime=inf
  LoaSt : Outport
  wires:
  Enumerated Constant/1 -> LoaSt/1

== system SF049A_LoaMgr/LoaMgr/LoaMgrPer1/Arbitrate_Responses/SelFinalResp/Norm ==
  F2 : ActionPort  ActionType=case
  CopyRight2 : Subsystem  Description=|  mask(Copyright Information){none=on}
      | Copyright info block.                                               
      |                                                                     
      | Place copyright information at the top of every subsystem in design.
      mask prompts: none "No parameters"
      mask help: Place copyright information at the top of every subsystem in design.
      mask Display:
      | NxtrConf = 'Nexteer Confidential';
      | 
      | sys = bdroot; %handle for the current model ("system")
      | first = get_param(sys,'Created');
      | first = first(end-3:end);  %year is last four digits
      | 
      | last = get_param(sys,'LastModifiedDate');
      | if isempty(last)
      |     last = datestr(now,'yyyy');
      | else
      |     last = last(end-3:end);
      | end
      | 
      | if strcmp(first,last)
      |     fprintf('%s -- Copyright %s Nexteer',NxtrConf,first)
      | else
      |     fprintf('%s -- %s%s- %s Nexteer',NxtrConf,char(169),first,last)
      | end
  Enumerated Constant : simulink/Sources/Enumerated Constant  OutDataTypeStr=Enum: LoaSt1  Value=LoaSt1.LOAST_NORM  SampleTime=inf
  LoaSt : Outport
  wires:
  Enumerated Constant/1 -> LoaSt/1

== system SF049A_LoaMgr/LoaMgr/LoaMgrPer1/Arbitrate_Responses/SelFinalResp/Reduced ==
  F2 : ActionPort  ActionType=case
  CopyRight2 : Subsystem  Description=|  mask(Copyright Information){none=on}
      | Copyright info block.                                               
      |                                                                     
      | Place copyright information at the top of every subsystem in design.
      mask prompts: none "No parameters"
      mask help: Place copyright information at the top of every subsystem in design.
      mask Display:
      | NxtrConf = 'Nexteer Confidential';
      | 
      | sys = bdroot; %handle for the current model ("system")
      | first = get_param(sys,'Created');
      | first = first(end-3:end);  %year is last four digits
      | 
      | last = get_param(sys,'LastModifiedDate');
      | if isempty(last)
      |     last = datestr(now,'yyyy');
      | else
      |     last = last(end-3:end);
      | end
      | 
      | if strcmp(first,last)
      |     fprintf('%s -- Copyright %s Nexteer',NxtrConf,first)
      | else
      |     fprintf('%s -- %s%s- %s Nexteer',NxtrConf,char(169),first,last)
      | end
  Enumerated Constant : simulink/Sources/Enumerated Constant  OutDataTypeStr=Enum: LoaSt1  Value=LoaSt1.LOAST_LIMD  SampleTime=inf
  LoaSt : Outport
  wires:
  Enumerated Constant/1 -> LoaSt/1

== system SF049A_LoaMgr/LoaMgr/LoaMgrPer1/Arbitrate_Responses/SelFinalResp/SwBasd_Mtgtn ==
  F2 : ActionPort  ActionType=case
  CopyRight2 : Subsystem  Description=|  mask(Copyright Information){none=on}
      | Copyright info block.                                               
      |                                                                     
      | Place copyright information at the top of every subsystem in design.
      mask prompts: none "No parameters"
      mask help: Place copyright information at the top of every subsystem in design.
      mask Display:
      | NxtrConf = 'Nexteer Confidential';
      | 
      | sys = bdroot; %handle for the current model ("system")
      | first = get_param(sys,'Created');
      | first = first(end-3:end);  %year is last four digits
      | 
      | last = get_param(sys,'LastModifiedDate');
      | if isempty(last)
      |     last = datestr(now,'yyyy');
      | else
      |     last = last(end-3:end);
      | end
      | 
      | if strcmp(first,last)
      |     fprintf('%s -- Copyright %s Nexteer',NxtrConf,first)
      | else
      |     fprintf('%s -- %s%s- %s Nexteer',NxtrConf,char(169),first,last)
      | end
  Enumerated Constant : simulink/Sources/Enumerated Constant  OutDataTypeStr=Enum: LoaSt1  Value=LoaSt1.LOAST_SWBASDMTGTN  SampleTime=inf
  LoaSt : Outport
  wires:
  Enumerated Constant/1 -> LoaSt/1

== system SF049A_LoaMgr/LoaMgr/LoaMgrPer1/Assign_Scale/F1/CopyRight2 ==

== system SF049A_LoaMgr/LoaMgr/LoaMgrPer1/Assign_Scale/F2/CopyRight2 ==

== system SF049A_LoaMgr/LoaMgr/LoaMgrPer1/Assign_Scale/Fade/CopyRight2 ==

== system SF049A_LoaMgr/LoaMgr/LoaMgrPer1/Assign_Scale/Limd/CopyRight2 ==

== system SF049A_LoaMgr/LoaMgr/LoaMgrPer1/Assign_Scale/Norm/CopyRight2 ==

== system SF049A_LoaMgr/LoaMgr/LoaMgrPer1/Assign_Scale/SwMtgtn/CopyRight2 ==

== system SF049A_LoaMgr/LoaMgr/LoaMgrPer1/Assign_Scale/SwMtgtn/HwTqTrue ==
  Action Port : ActionPort  ActionType=then
  Constant1 : Constant  RequirementInfo="{'linktype_rmi_doors' '0000bab3 (/E-STEER Core/SubSystem Specifications/Application Functions/SF049A Loss of Assist Manager)' '#SF049A_99' 'true' 'REQ:  SF049A_99' '' } %GIDa_1c7a28f8_e99d_4d23_82aa_c24fb5cec3da"  Value=LOAMAXSLEW_ULSPERSEC_F32
  Constant6 : Constant  RequirementInfo="{'linktype_rmi_doors' '0000bab3 (/E-STEER Core/SubSystem Specifications/Application Functions/SF049A Loss of Assist Manager)' '#SF049A_99' 'true' 'REQ:  SF049A_99' '' } %GIDa_ade64fcd_95c6_4c96_abc7_ff6dd867402d"  Value=LOASCAONE_ULS_F32
  CopyRight2 : Subsystem  Description=|  mask(Copyright Information){none=on}
      | Copyright info block.                                               
      |                                                                     
      | Place copyright information at the top of every subsystem in design.
      mask prompts: none "No parameters"
      mask help: Place copyright information at the top of every subsystem in design.
      mask Display:
      | NxtrConf = 'Nexteer Confidential';
      | 
      | sys = bdroot; %handle for the current model ("system")
      | first = get_param(sys,'Created');
      | first = first(end-3:end);  %year is last four digits
      | 
      | last = get_param(sys,'LastModifiedDate');
      | if isempty(last)
      |     last = datestr(now,'yyyy');
      | else
      |     last = last(end-3:end);
      | end
      | 
      | if strcmp(first,last)
      |     fprintf('%s -- Copyright %s Nexteer',NxtrConf,first)
      | else
      |     fprintf('%s -- %s%s- %s Nexteer',NxtrConf,char(169),first,last)
      | end
  Sca : Outport  RequirementInfo="{'linktype_rmi_doors' '0000bab3 (/E-STEER Core/SubSystem Specifications/Application Functions/SF049A Loss of Assist Manager)' '#SF049A_99' 'true' 'REQ:  SF049A_99' '' } %GIDa_010c1524_9c3d_4e76_85cf_da1fff0532cd"
  Rate : Outport  RequirementInfo="{'linktype_rmi_doors' '0000bab3 (/E-STEER Core/SubSystem Specifications/Application Functions/SF049A Loss of Assist Manager)' '#SF049A_99' 'true' 'REQ:  SF049A_99' '' } %GIDa_abd8b895_2dca_4b35_9b2e_3545e82a9dc9"  Port=2
  wires:
  Constant6/1 -> Sca/1
  Constant1/1 -> Rate/1
